simulink model "Quadcopter_LQR_with_noise"  (R2022a)
settings: Solver=VariableStepAuto  StartTime=0.0  StopTime=10.0  RelTol=1e-3
values from neighbouring files (symbols this model uses):
  A_mat = [0 0 0 0 0 0 1 0 0 0 0 0 ... (first row only)    [initialquadt.m]
  B_mat = [ ... (first row only)    [initialquadt.m]
  C_mat = eye(12)    [initialquadt.m]
  K_mat = lqr(A_mat,B_mat,Q_mat,R_mat)    [initialquadt.m]
libraries: simulink x1
settings Model: Creator=HP  LastModifiedBy=HP

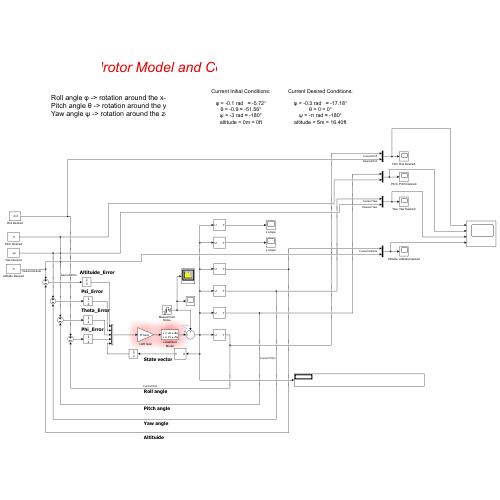
[thumbnail: Simulink's stored preview of the top-level diagram]
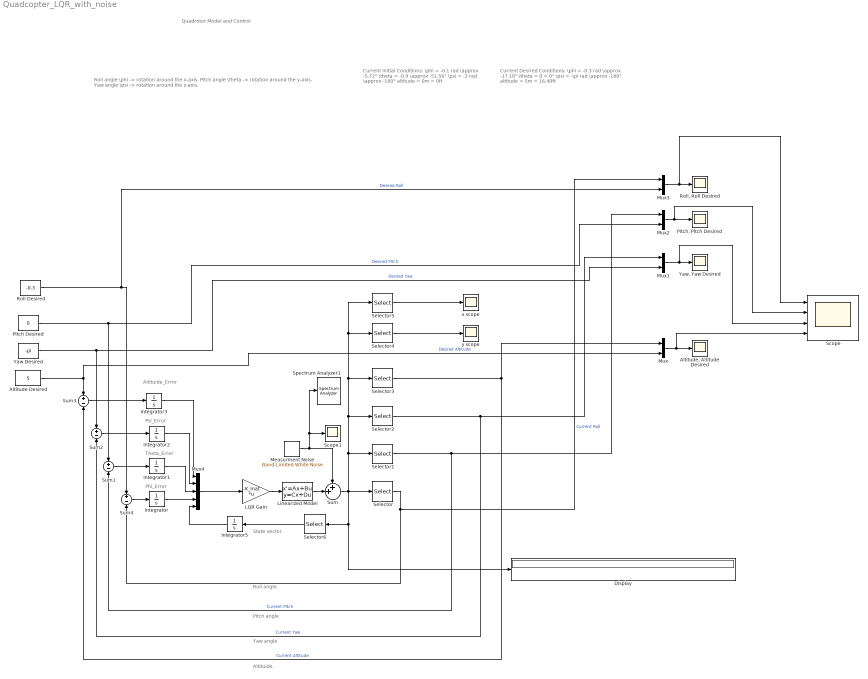
== system Quadcopter_LQR_with_noise ==
  note: Current Initial Conditions:
      |
      | \phi = -0.1 rad   \approx -5.72°
      | \theta = -0.9 \approx -51.56°
      | \psi = -3 rad \approx -180°
      | altitude = 0m = 0ft
  note: Roll angle \phi -> rotation around the x-axis.
      | Pitch angle \theta -> rotation around the y-axis.
      | Yaw angle \psi -> rotation around the z-axis.
  note: State vector
  note: Current Desired Conditions:
      |
      | \phi = -0.3 rad   \approx -17.18°
      | \theta = 0 = 0°
      | \psi = -\pi rad \approx -180°
      | altitude = 5m = 16.40ft
  note: Quadrotor Model and Control
  note: Altituide_Error
  note: Phi_Error
  note: Psi_Error
  note: Pitch angle
  note: Yaw angle
  note: Roll angle
  note: Theta_Error
  note: Altituide
  Altitude Desired : Constant  Value=5
  "Altitude, Altitude Desired" : Scope
  Display : Display
  Integrator : Integrator  InitialCondition=-0.1
  Integrator1 : Integrator  InitialCondition=-0.9
  Integrator2 : Integrator  InitialCondition=-3
  Integrator3 : Integrator
  Integrator5 : Integrator
  LQR Gain : Gain  Gain=-K_mat  Multiplication=Matrix(K*u) (u vector)  SaturateOnIntegerOverflow=on  OutDataTypeStr=Inherit: Same as input  ParamDataTypeStr=Inherit: Same as input
  Linearized Model : StateSpace  A=A_mat-B_mat*K_mat  B=B_mat  C=C_mat  D=zeros(12,4)  InitialCondition=0
  Measurment Noise : simulink/Sources/Band-Limited White Noise  Cov=[0.00005]  Ts=0.0001  seed=[23341]
  Mux{,1..3} (4 alike) : Mux  Inputs=2
  Mux4 : Mux  Inputs=5
  Pitch Desired : Constant  Value=0
  "Pitch, Pitch Desired" : Scope
  Roll Desired : Constant  Value=-0.3
  "Roll, Roll Desired" : Scope
  Scope : Scope  NumInputPorts=4
  Scope1 : Scope
  Selector : Selector  InputPortWidth=12  IndexOptions=Index vector (dialog)  Indices=[1]  OutputSizes=1
  Selector1 : Selector  InputPortWidth=12  IndexOptions=Index vector (dialog)  Indices=[2]  OutputSizes=1
  Selector2 : Selector  InputPortWidth=12  IndexOptions=Index vector (dialog)  Indices=[3]  OutputSizes=1
  Selector3 : Selector  InputPortWidth=12  IndexOptions=Index vector (dialog)  Indices=[6]  OutputSizes=1
  Selector4 : Selector  InputPortWidth=12  IndexOptions=Index vector (dialog)  Indices=[5]  OutputSizes=1
  Selector5 : Selector  InputPortWidth=12  IndexOptions=Index vector (dialog)  Indices=[4]  OutputSizes=1
  Selector6 : Selector  InputPortWidth=12  IndexOptions=Index vector (dialog)  Indices=[4 5 7 :12]  OutputSizes=1
  Spectrum Analyzer1 : SpectrumAnalyzer
  Sum : Sum  Inputs=++|
  Sum{1..4} (4 alike) : Sum  Inputs=+-  InputSameDT=on  SaturateOnIntegerOverflow=on  OutDataTypeStr=Inherit: Same as first input
  Yaw Desired : Constant  Value=-pi
  "Yaw, Yaw Desired" : Scope
  x scope : Scope
  y scope : Scope
  wires:
  LQR Gain/1 -> Linearized Model/1
  Measurment Noise/1 -> Spectrum Analyzer1/1, Scope1/1, Sum/1
  Yaw Desired/1 -> Mux1/2, Sum2/1  "Desired Yaw"
  Sum3/1 -> Integrator3/1
  Selector6/1 -> Integrator5/1
  Selector1/1 -> Mux2/1, Sum1/2  "Current Pitch"
  Pitch Desired/1 -> Mux2/2, Sum1/1  "Desired Pitch"
  Sum/1 -> Selector3/1, Selector5/1, Selector4/1, Selector2/1, Selector1/1, Display/1, Selector6/1, Selector/1
  Mux/1 -> Scope/4, "Altitude, Altitude Desired"/1
  Integrator3/1 -> Mux4/1
  Sum4/1 -> Integrator/1
  Roll Desired/1 -> Sum4/1, Mux3/2  "Desired Roll"
  Selector4/1 -> y scope/1
  Selector2/1 -> Mux1/1, Sum2/2  "Current Yaw"
  Selector5/1 -> x scope/1
  Integrator2/1 -> Mux4/2
  Sum2/1 -> Integrator2/1
  Sum1/1 -> Integrator1/1
  Altitude Desired/1 -> Mux/2, Sum3/1  "Desired Altitude"
  Mux2/1 -> Scope/2, "Pitch, Pitch Desired"/1
  Selector/1 -> Mux3/1, Sum4/2  "Current Roll"
  Integrator5/1 -> Mux4/5
  Selector3/1 -> Sum3/2, Mux/1  "Current Altitude"
  Linearized Model/1 -> Sum/2
  Mux4/1 -> LQR Gain/1
  Integrator1/1 -> Mux4/3
  Mux3/1 -> Scope/1, "Roll, Roll Desired"/1
  Mux1/1 -> Scope/3, "Yaw, Yaw Desired"/1
  Integrator/1 -> Mux4/4
